simulink model "Cruise_Control"  (R2020a)
settings: Solver=VariableStepAuto  StartTime=0.0  StopTime=10.0  RelTol=1e-3
values from neighbouring files (symbols this model uses):
  Ki = 1    [Cruise_Control.mat]
  Kp = 1    [Cruise_Control.mat]
settings Model: Creator=kapfumv  LastModifiedBy=kapfumv

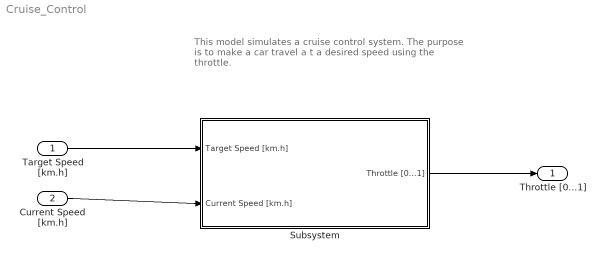
== system Cruise_Control ==
  note: This model simulates a cruise control system.
      | The purpose is to make a car travel a t a desired speed
      | using the throttle.
  Target Speed [km.h] : Inport
  Current Speed [km.h] : Inport  Port=2
  Subsystem : Subsystem
  Throttle [0...1] : Outport
  wires:
  Target Speed [km.h]/1 -> Subsystem/1(Target Speed [km.h])
  Current Speed [km.h]/1 -> Subsystem/2(Current Speed [km.h])
  Subsystem/1(Throttle [0...1]) -> Throttle [0...1]/1

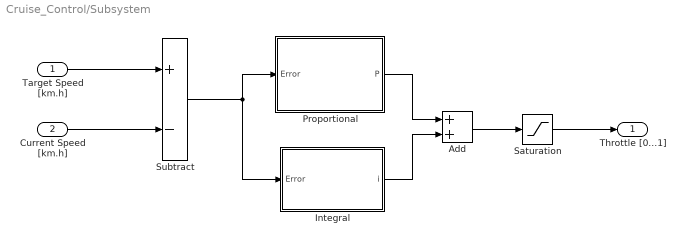
== system Cruise_Control/Subsystem ==
  Target Speed [km.h] : Inport
  Current Speed [km.h] : Inport  Port=2
  Add : Sum
  Integral : Subsystem
  Proportional : Subsystem
  Saturation : Saturate
  Subtract : Sum  Inputs=+-
  Throttle [0...1] : Outport
  wires:
  Integral/1(i) -> Add/2
  Add/1 -> Saturation/1
  Target Speed [km.h]/1 -> Subtract/1
  Proportional/1(P) -> Add/1
  Subtract/1 -> Integral/1(Error), Proportional/1(Error)
  Saturation/1 -> Throttle [0...1]/1
  Current Speed [km.h]/1 -> Subtract/2

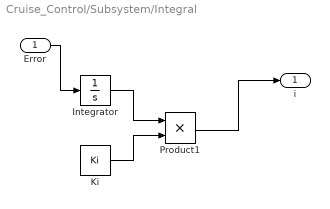
== system Cruise_Control/Subsystem/Integral ==
  Error : Inport
  Integrator : Integrator
  Ki : Constant  Value=Ki
  Product1 : Product
  i : Outport
  wires:
  Integrator/1 -> Product1/1
  Ki/1 -> Product1/2
  Product1/1 -> i/1
  Error/1 -> Integrator/1

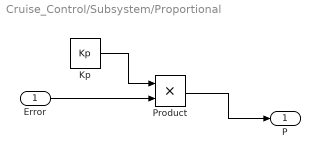
== system Cruise_Control/Subsystem/Proportional ==
  Error : Inport
  Kp : Constant  Value=Kp
  Product : Product
  P : Outport
  wires:
  Product/1 -> P/1
  Kp/1 -> Product/1
  Error/1 -> Product/2
